simulink model "FuelT_DD"  (R2016b)
settings: configuration reference "CodeGenConfigSet" (kept outside this file)
values from neighbouring files (symbols this model uses):
  FuelT_swtTempPlaSel_C = Calibration.Parameter    [init_FuelT_DD.m]
  FuelT_tDiffMaxHi_C = Calibration.Parameter    [init_FuelT_DD.m]
  FuelT_tDiffMaxLo_C = Calibration.Parameter    [init_FuelT_DD.m]
  FuelT_tiMaxDefDeb_C = Calibration.Parameter    [init_FuelT_DD.m]
  FuelT_tiMaxOKDeb_C = Calibration.Parameter    [init_FuelT_DD.m]
  FuelT_tiMinDefDeb_C = Calibration.Parameter    [init_FuelT_DD.m]
  FuelT_tiMinOKDeb_C = Calibration.Parameter    [init_FuelT_DD.m]
  FuelT_tiPlausHiDefDeb_C = Calibration.Parameter    [init_FuelT_DD.m]
  FuelT_tiPlausHiOKDeb_C = Calibration.Parameter    [init_FuelT_DD.m]
  FuelT_tiPlausLoDefDeb_C = Calibration.Parameter    [init_FuelT_DD.m]
  FuelT_tiPlausLoOKDeb_C = Calibration.Parameter    [init_FuelT_DD.m]
  FuelT_tTransf_CUR = Calibration.Parameter    [init_FuelT_DD.m]
  FuelT_tTransf_CURX = Calibration.Parameter    [init_FuelT_DD.m]
  FuelT_uSRCMax_C = Calibration.Parameter    [init_FuelT_DD.m]
  FuelT_uSRCMin_C = Calibration.Parameter    [init_FuelT_DD.m]
undefined symbols (not defined in the file or in its folder): CEngDsT_tTransf_CURX, FuelT_DD_DT, Switch_conv
libraries: CXLib x12
settings Model: Creator=Wollf  LastModifiedBy=wangrui
settings ConfigSetRef: SourceLocation=Base Workspace

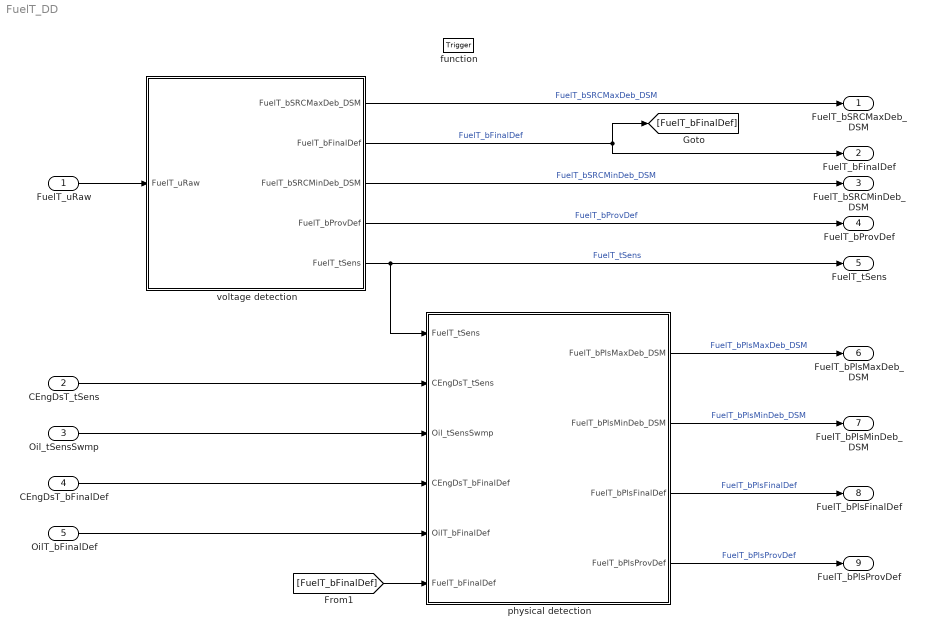
== system FuelT_DD ==
  FuelT_uRaw : Inport  Tag=mv  Description=Raw ADC value of fuel temperature  OutMin=0  OutMax=5000  OutDataTypeStr=Ad_mv
  CEngDsT_tSens : Inport  Tag=deg  Description=Sensed engine coolant temperature  Port=2  OutMin=-200  OutMax=200  OutDataTypeStr=Temp_deg
  Oil_tSensSwmp : Inport  Tag=deg  Description=Sensed value of oil temperature  Port=3  OutMin=-50  OutMax=200  OutDataTypeStr=Temp_deg
  CEngDsT_bFinalDef : Inport  Description=Status Sensor of the coolant temperature finally defect  Port=4  OutMin=0  OutMax=1  OutDataTypeStr=boolean
  OilT_bFinalDef : Inport  Description=Status Sensor of the oil temperature finally defect  Port=5  OutMin=0  OutMax=1  OutDataTypeStr=boolean
  function : TriggerPort  TriggerType=function-call  VariantControl=Variant
  physical detection : Subsystem
  voltage detection : Subsystem
  FuelT_bSRCMaxDeb_DSM : Outport  Description=status of FuelT_bSRCMaxDeb  OutMin=0  OutMax=1  OutDataTypeStr=boolean
  FuelT_bFinalDef : Outport  Description=Status sensor of the fuel temperature finally defect  Port=2  OutMin=0  OutMax=1  OutDataTypeStr=boolean
  FuelT_bSRCMinDeb_DSM : Outport  Description=status of FuelT_bSRCMinDeb  Port=3  OutMin=0  OutMax=1  OutDataTypeStr=boolean
  FuelT_bProvDef : Outport  Description=Status sensor of the fuel temperature temporary defect  Port=4  OutMin=0  OutMax=1  OutDataTypeStr=boolean
  FuelT_tSens : Outport  Tag=deg  Description=Sensed fuel temperature  Port=5  OutMin=-50  OutMax=150  OutDataTypeStr=Temp_deg
  FuelT_bPlsMaxDeb_DSM : Outport  Description=status of FuelT_bPlsMaxDeb  Port=6  OutMin=0  OutMax=1  OutDataTypeStr=boolean
  FuelT_bPlsMinDeb_DSM : Outport  Description=status of FuelT_bPlsMinDeb  Port=7  OutMin=0  OutMax=1  OutDataTypeStr=boolean
  FuelT_bPlsFinalDef : Outport  Description=Status sensor of the fuel temperature physical signal range check finally defect  Port=8  OutMin=0  OutMax=1  OutDataTypeStr=boolean
  FuelT_bPlsProvDef : Outport  Description=Status sensor of the fuel temperature physical signal range check temporary defect  Port=9  OutMin=0  OutMax=1  OutDataTypeStr=boolean
  wires:
  FuelT_uRaw/1 -> voltage detection/1(FuelT_uRaw)
  voltage detection/1(FuelT_bSRCMaxDeb_DSM) -> FuelT_bSRCMaxDeb_DSM/1  "FuelT_bSRCMaxDeb_DSM"
  voltage detection/2(FuelT_bFinalDef) -> FuelT_bFinalDef/1, [FuelT_bFinalDef]  "FuelT_bFinalDef"
  voltage detection/3(FuelT_bSRCMinDeb_DSM) -> FuelT_bSRCMinDeb_DSM/1  "FuelT_bSRCMinDeb_DSM"
  voltage detection/4(FuelT_bProvDef) -> FuelT_bProvDef/1  "FuelT_bProvDef"
  voltage detection/5(FuelT_tSens) -> FuelT_tSens/1, physical detection/1(FuelT_tSens)  "FuelT_tSens"
  CEngDsT_tSens/1 -> physical detection/2(CEngDsT_tSens)
  Oil_tSensSwmp/1 -> physical detection/3(Oil_tSensSwmp)
  CEngDsT_bFinalDef/1 -> physical detection/4(CEngDsT_bFinalDef)
  OilT_bFinalDef/1 -> physical detection/5(OilT_bFinalDef)
  physical detection/1(FuelT_bPlsMaxDeb_DSM) -> FuelT_bPlsMaxDeb_DSM/1  "FuelT_bPlsMaxDeb_DSM"
  physical detection/2(FuelT_bPlsMinDeb_DSM) -> FuelT_bPlsMinDeb_DSM/1  "FuelT_bPlsMinDeb_DSM"
  physical detection/3(FuelT_bPlsFinalDef) -> FuelT_bPlsFinalDef/1  "FuelT_bPlsFinalDef"
  physical detection/4(FuelT_bPlsProvDef) -> FuelT_bPlsProvDef/1  "FuelT_bPlsProvDef"
  [FuelT_bFinalDef] -> physical detection/6(FuelT_bFinalDef)

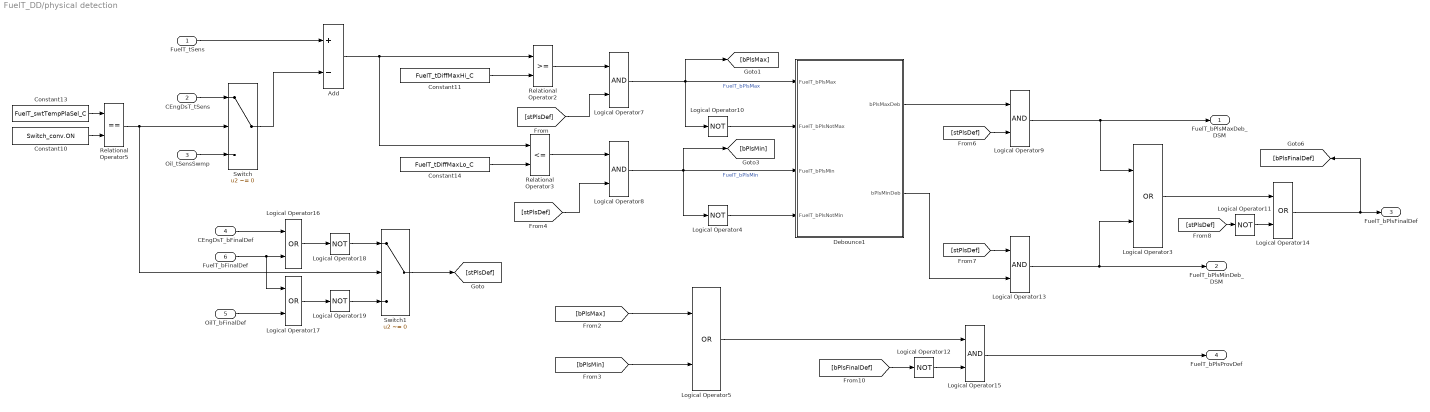
== system FuelT_DD/physical detection ==
  FuelT_tSens : Inport
  CEngDsT_tSens : Inport  Tag=deg  Description=Sensed engine coolant temperature  Port=2  OutMin=-50  OutMax=150  OutDataTypeStr=Temp_deg
  Oil_tSensSwmp : Inport  Tag=deg  Description=Sensed engine oil temperature  Port=3  OutMin=-50  OutMax=200  OutDataTypeStr=Temp_deg
  CEngDsT_bFinalDef : Inport  Tag=-  Description=Status Sensor of the coolant temperature finally defect  Port=4  OutMin=0  OutMax=1  OutDataTypeStr=boolean
  OilT_bFinalDef : Inport  Tag=-  Description=Status Sensor of the oil temperature finally defect  Port=5  OutMin=0  OutMax=1  OutDataTypeStr=boolean
  FuelT_bFinalDef : Inport  Port=6
  Add : Sum  Inputs=+-  OutDataTypeStr=Inherit: Inherit via back propagation  InputSameDT=on
  Constant10 : Constant  Value=Switch_conv.ON  OutDataTypeStr=Inherit: Inherit via back propagation
  Constant11 : Constant  Value=FuelT_tDiffMaxHi_C
  Constant13 : Constant  Value=FuelT_swtTempPlaSel_C  SampleTime=-1
  Constant14 : Constant  Value=FuelT_tDiffMaxLo_C
  Debounce1 : Subsystem
  Logical Operator{4,10..12,18..19} (6 alike) : Logic  Operator=NOT  AllPortsSameDT=off  OutDataTypeStr=boolean
  Logical Operator{7..9,13,15} (5 alike) : Logic  AllPortsSameDT=off  OutDataTypeStr=boolean
  Logical Operator{3,5,14,16..17} (5 alike) : Logic  Operator=OR  AllPortsSameDT=off  OutDataTypeStr=boolean
  Relational Operator2 : RelationalOperator  OutDataTypeStr=boolean  RndMeth=Nearest  InputSameDT=on
  Relational Operator3 : RelationalOperator  Operator=<=  OutDataTypeStr=boolean  RndMeth=Nearest  InputSameDT=on
  Relational Operator5 : RelationalOperator  Operator===  OutDataTypeStr=boolean  RndMeth=Simplest  InputSameDT=on
  Switch : Switch  Criteria=u2 ~= 0  InputSameDT=on
  Switch1 : Switch  Criteria=u2 ~= 0  InputSameDT=on
  FuelT_bPlsMaxDeb_DSM : Outport  Tag=-  Description=status of FuelT_bPlsMaxDeb  OutMin=0  OutMax=1  OutDataTypeStr=boolean
  FuelT_bPlsMinDeb_DSM : Outport  Tag=-  Description=status of FuelT_bPlsMinDeb  Port=2  OutMin=0  OutMax=1  OutDataTypeStr=boolean
  FuelT_bPlsFinalDef : Outport  Tag=-  Description=Status sensor of the fuel temperature physical signal range check finally defect  Port=3  OutMin=0  OutMax=1  OutDataTypeStr=boolean
  FuelT_bPlsProvDef : Outport  Tag=-  Description=Status sensor of the coolant temperature physical signal range check temporary defect  Port=4  OutMin=0  OutMax=1  OutDataTypeStr=boolean
  wires:
  FuelT_tSens/1 -> Add/1
  Constant13/1 -> Relational Operator5/1
  Constant10/1 -> Relational Operator5/2
  Relational Operator5/1 -> Switch1/2, Switch/2
  CEngDsT_tSens/1 -> Switch/1
  Oil_tSensSwmp/1 -> Switch/3
  Switch/1 -> Add/2
  Add/1 -> Relational Operator3/1, Relational Operator2/1
  Constant11/1 -> Relational Operator2/2
  Logical Operator7/1 -> Logical Operator10/1, [bPlsMax], Debounce1/1(FuelT_bPlsMax)  "FuelT_bPlsMax"
  Constant14/1 -> Relational Operator3/2
  Logical Operator8/1 -> Logical Operator4/1, [bPlsMin], Debounce1/3(FuelT_bPlsMin)  "FuelT_bPlsMin"
  Logical Operator9/1 -> FuelT_bPlsMaxDeb_DSM/1, Logical Operator3/1
  Logical Operator13/1 -> FuelT_bPlsMinDeb_DSM/1, Logical Operator3/2
  [bPlsMax] -> Logical Operator5/1
  [bPlsMin] -> Logical Operator5/2
  Relational Operator2/1 -> Logical Operator7/1
  [stPlsDef] -> Logical Operator7/2
  Relational Operator3/1 -> Logical Operator8/1
  [stPlsDef] -> Logical Operator8/2
  [stPlsDef] -> Logical Operator9/2
  [stPlsDef] -> Logical Operator13/1
  Logical Operator3/1 -> Logical Operator14/1
  [stPlsDef] -> Logical Operator11/1
  Logical Operator14/1 -> [bPlsFinalDef], FuelT_bPlsFinalDef/1
  Logical Operator15/1 -> FuelT_bPlsProvDef/1
  Logical Operator11/1 -> Logical Operator14/2
  Logical Operator10/1 -> Debounce1/2(FuelT_bPlsNotMax)
  Logical Operator4/1 -> Debounce1/4(FuelT_bPlsNotMin)
  Debounce1/1(bPlsMaxDeb) -> Logical Operator9/1
  Debounce1/2(bPlsMinDeb) -> Logical Operator13/2
  FuelT_bFinalDef/1 -> Logical Operator17/1, Logical Operator16/2
  CEngDsT_bFinalDef/1 -> Logical Operator16/1
  Logical Operator16/1 -> Logical Operator18/1
  Logical Operator17/1 -> Logical Operator19/1
  OilT_bFinalDef/1 -> Logical Operator17/2
  Switch1/1 -> [stPlsDef]
  Logical Operator18/1 -> Switch1/1
  Logical Operator19/1 -> Switch1/3
  [bPlsFinalDef] -> Logical Operator12/1
  Logical Operator12/1 -> Logical Operator15/2
  Logical Operator5/1 -> Logical Operator15/1

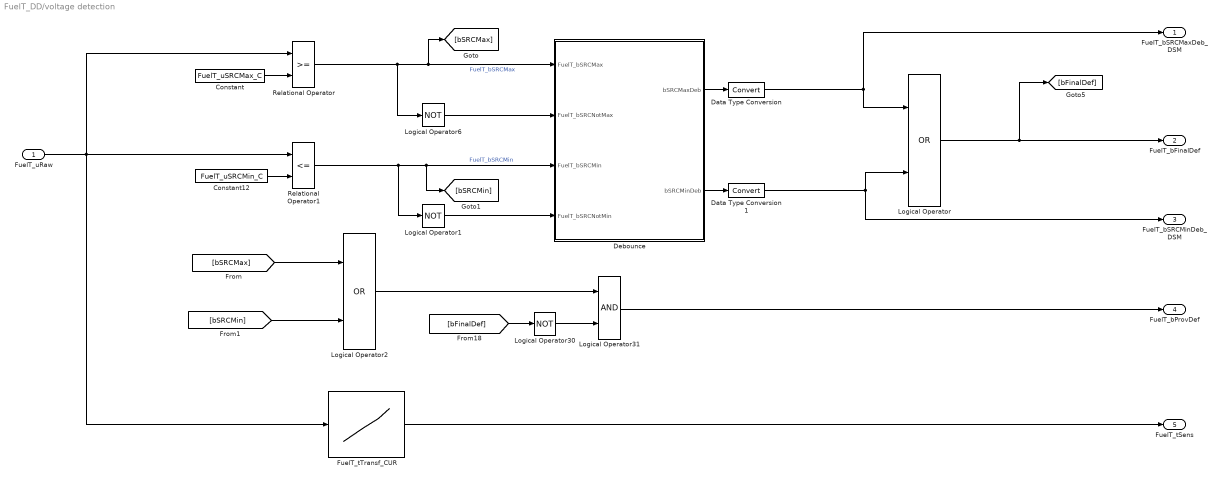
== system FuelT_DD/voltage detection ==
  FuelT_uRaw : Inport  Tag=mv  Description=Raw ADC value of fuel temperature  OutMin=0  OutMax=5000  OutDataTypeStr=Ad_mv
  Constant : Constant  Value=FuelT_uSRCMax_C
  Constant12 : Constant  Value=FuelT_uSRCMin_C
  Data Type Conversion : DataTypeConversion
  Data Type Conversion1 : DataTypeConversion
  Debounce : Subsystem
  FuelT_tTransf_CUR : Lookup_n-D  DialogController=Simulink.DDGSource  NumberOfTableDimensions=1  BreakpointsForDimension1=FuelT_tTransf_CURX  BreakpointsForDimension2=CEngDsT_tTransf_CURX  IndexSearchMethod=Linear search  BeginIndexSearchUsingPreviousIndexResult=on  Table=FuelT_tTransf_CUR  ExtrapMethod=Clip  UseLastTableValue=on  InternalRulePriority=Speed  OutDataTypeStr=Inherit: Inherit via back propagation  SaturateOnIntegerOverflow=on
  Logical Operator : Logic  Operator=OR  AllPortsSameDT=off  OutDataTypeStr=boolean
  Logical Operator1 : Logic  Operator=NOT  AllPortsSameDT=off  OutDataTypeStr=boolean
  Logical Operator2 : Logic  Operator=OR  AllPortsSameDT=off  OutDataTypeStr=boolean
  Logical Operator30 : Logic  Operator=NOT  AllPortsSameDT=off  OutDataTypeStr=boolean
  Logical Operator31 : Logic  AllPortsSameDT=off  OutDataTypeStr=boolean
  Logical Operator6 : Logic  Operator=NOT  AllPortsSameDT=off  OutDataTypeStr=boolean
  Relational Operator : RelationalOperator  OutDataTypeStr=boolean  RndMeth=Nearest  InputSameDT=on
  Relational Operator1 : RelationalOperator  Operator=<=  OutDataTypeStr=boolean  RndMeth=Nearest  InputSameDT=on
  FuelT_bSRCMaxDeb_DSM : Outport  Tag=-  Description=status of FuelT_bSRCMaxDeb  OutMin=0  OutMax=1  OutDataTypeStr=boolean
  FuelT_bFinalDef : Outport  Tag=-  Description=Status sensor of the fuel temperature finally defect  Port=2  OutMin=0  OutMax=1  OutDataTypeStr=boolean
  FuelT_bSRCMinDeb_DSM : Outport  Tag=-  Description=status of FuelT_bSRCMinDeb  Port=3  OutMin=0  OutMax=1  OutDataTypeStr=boolean
  FuelT_bProvDef : Outport  Tag=-  Description=Status sensor of the fuel temperature temporary defect  Port=4  OutMin=0  OutMax=1  OutDataTypeStr=boolean
  FuelT_tSens : Outport  Tag=-  Description=Sensed fuel temperature  Port=5  OutMin=-50  OutMax=150  OutDataTypeStr=Temp_deg
  wires:
  FuelT_tTransf_CUR/1 -> FuelT_tSens/1
  FuelT_uRaw/1 -> FuelT_tTransf_CUR/1, Relational Operator/1, Relational Operator1/1
  Constant/1 -> Relational Operator/2
  Relational Operator/1 -> Logical Operator6/1, [bSRCMax], Debounce/1(FuelT_bSRCMax)  "FuelT_bSRCMax"
  Constant12/1 -> Relational Operator1/2
  Relational Operator1/1 -> Logical Operator1/1, [bSRCMin], Debounce/3(FuelT_bSRCMin)  "FuelT_bSRCMin"
  Debounce/1(bSRCMaxDeb) -> Data Type Conversion/1
  Debounce/2(bSRCMinDeb) -> Data Type Conversion1/1
  [bSRCMax] -> Logical Operator2/1
  [bSRCMin] -> Logical Operator2/2
  Logical Operator/1 -> FuelT_bFinalDef/1, [bFinalDef]
  Logical Operator6/1 -> Debounce/2(FuelT_bSRCNotMax)
  Logical Operator1/1 -> Debounce/4(FuelT_bSRCNotMin)
  Data Type Conversion/1 -> FuelT_bSRCMaxDeb_DSM/1, Logical Operator/1
  Data Type Conversion1/1 -> FuelT_bSRCMinDeb_DSM/1, Logical Operator/2
  [bFinalDef] -> Logical Operator30/1
  Logical Operator30/1 -> Logical Operator31/2
  Logical Operator2/1 -> Logical Operator31/1
  Logical Operator31/1 -> FuelT_bProvDef/1

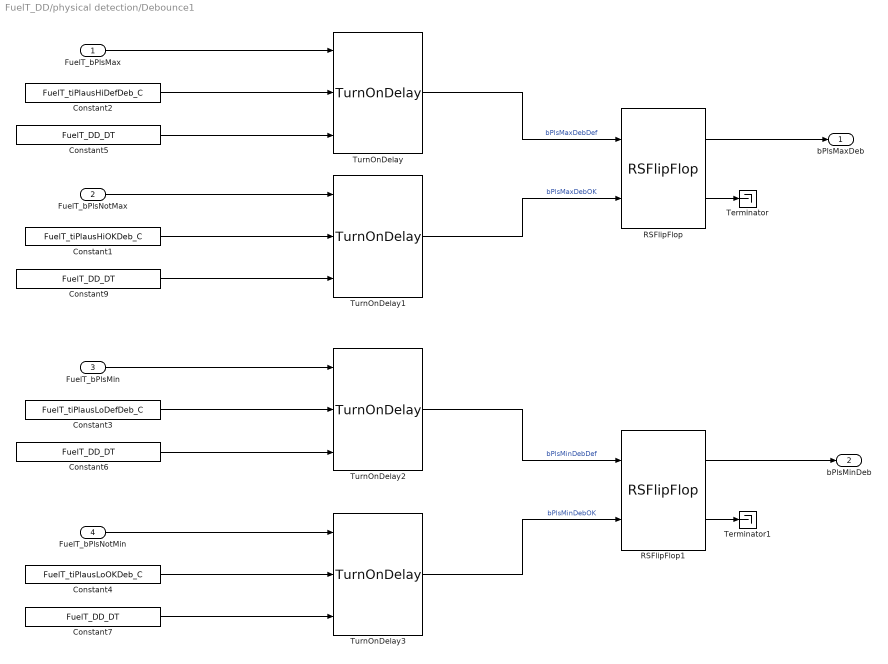
== system FuelT_DD/physical detection/Debounce1 ==
  FuelT_bPlsMax : Inport
  FuelT_bPlsNotMax : Inport  Port=2
  FuelT_bPlsMin : Inport  Port=3
  FuelT_bPlsNotMin : Inport  Port=4
  Constant1 : Constant  Value=FuelT_tiPlausHiOKDeb_C
  Constant2 : Constant  Value=FuelT_tiPlausHiDefDeb_C
  Constant3 : Constant  Value=FuelT_tiPlausLoDefDeb_C
  Constant4 : Constant  Value=FuelT_tiPlausLoOKDeb_C
  Constant{5..7,9} (4 alike) : Constant  Value=FuelT_DD_DT  OutDataTypeStr=Inherit: Inherit via back propagation
  RSFlipFlop : CXLib/RSFlipFlop
  RSFlipFlop1 : CXLib/RSFlipFlop
  Terminator : Terminator
  Terminator1 : Terminator
  TurnOnDelay{,1..3} (4 alike) : CXLib/TurnOnDelay
  bPlsMaxDeb : Outport
  bPlsMinDeb : Outport  Port=2
  wires:
  Constant7/1 -> TurnOnDelay3/3
  Constant6/1 -> TurnOnDelay2/3
  Constant9/1 -> TurnOnDelay1/3
  Constant5/1 -> TurnOnDelay/3
  FuelT_bPlsMax/1 -> TurnOnDelay/1
  RSFlipFlop1/2 -> Terminator1/1
  RSFlipFlop/2 -> Terminator/1
  Constant4/1 -> TurnOnDelay3/2
  TurnOnDelay3/1 -> RSFlipFlop1/2  "bPlsMinDebOK"
  FuelT_bPlsNotMin/1 -> TurnOnDelay3/1
  TurnOnDelay2/1 -> RSFlipFlop1/1  "bPlsMinDebDef"
  FuelT_bPlsMin/1 -> TurnOnDelay2/1
  FuelT_bPlsNotMax/1 -> TurnOnDelay1/1
  TurnOnDelay/1 -> RSFlipFlop/1  "bPlsMaxDebDef"
  Constant2/1 -> TurnOnDelay/2
  Constant1/1 -> TurnOnDelay1/2
  Constant3/1 -> TurnOnDelay2/2
  TurnOnDelay1/1 -> RSFlipFlop/2  "bPlsMaxDebOK"
  RSFlipFlop/1 -> bPlsMaxDeb/1
  RSFlipFlop1/1 -> bPlsMinDeb/1

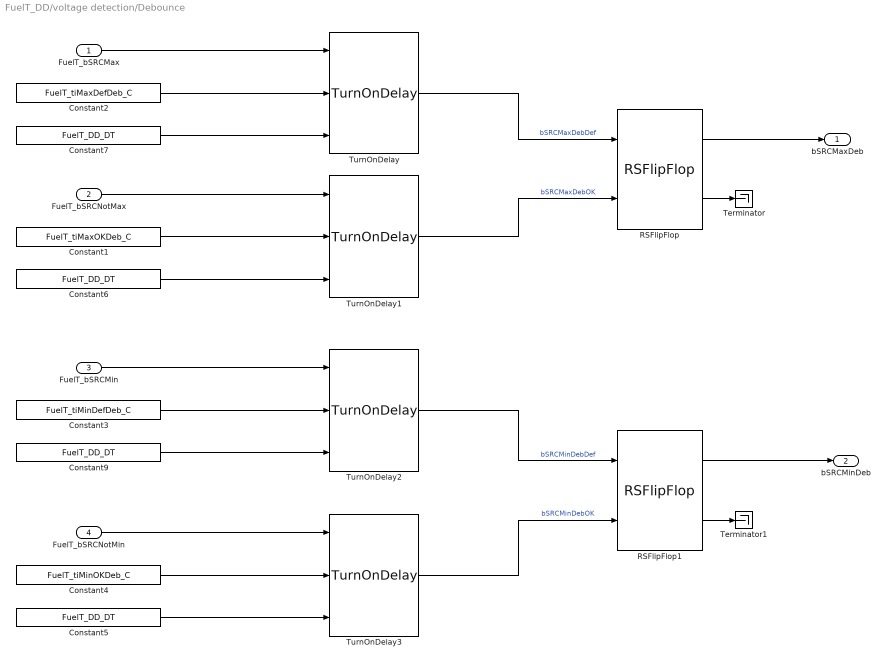
== system FuelT_DD/voltage detection/Debounce ==
  FuelT_bSRCMax : Inport
  FuelT_bSRCNotMax : Inport  Port=2
  FuelT_bSRCMin : Inport  Port=3
  FuelT_bSRCNotMin : Inport  Port=4
  Constant1 : Constant  Value=FuelT_tiMaxOKDeb_C
  Constant2 : Constant  Value=FuelT_tiMaxDefDeb_C
  Constant3 : Constant  Value=FuelT_tiMinDefDeb_C
  Constant4 : Constant  Value=FuelT_tiMinOKDeb_C
  Constant{5..7,9} (4 alike) : Constant  Value=FuelT_DD_DT  OutDataTypeStr=Inherit: Inherit via back propagation
  RSFlipFlop : CXLib/RSFlipFlop
  RSFlipFlop1 : CXLib/RSFlipFlop
  Terminator : Terminator
  Terminator1 : Terminator
  TurnOnDelay{,1..3} (4 alike) : CXLib/TurnOnDelay
  bSRCMaxDeb : Outport
  bSRCMinDeb : Outport  Port=2
  wires:
  Constant5/1 -> TurnOnDelay3/3
  Constant9/1 -> TurnOnDelay2/3
  Constant6/1 -> TurnOnDelay1/3
  Constant7/1 -> TurnOnDelay/3
  FuelT_bSRCMax/1 -> TurnOnDelay/1
  RSFlipFlop1/2 -> Terminator1/1
  RSFlipFlop/2 -> Terminator/1
  Constant4/1 -> TurnOnDelay3/2
  TurnOnDelay3/1 -> RSFlipFlop1/2  "bSRCMinDebOK"
  FuelT_bSRCNotMin/1 -> TurnOnDelay3/1
  TurnOnDelay2/1 -> RSFlipFlop1/1  "bSRCMinDebDef"
  FuelT_bSRCMin/1 -> TurnOnDelay2/1
  FuelT_bSRCNotMax/1 -> TurnOnDelay1/1
  TurnOnDelay/1 -> RSFlipFlop/1  "bSRCMaxDebDef"
  Constant2/1 -> TurnOnDelay/2
  Constant1/1 -> TurnOnDelay1/2
  Constant3/1 -> TurnOnDelay2/2
  TurnOnDelay1/1 -> RSFlipFlop/2  "bSRCMaxDebOK"
  RSFlipFlop/1 -> bSRCMaxDeb/1
  RSFlipFlop1/1 -> bSRCMinDeb/1
